simulink model "raspberrypi_sensehat_ev3robot"  (R2018b)
settings: Solver=FixedStepAuto  StartTime=0.0  StopTime=inf  RelTol=1e-3
libraries: sensehatlib x1, embdlinuxlib x1
settings Model: SimulationMode=external  Creator=The MathWorks, Inc.  LastModifiedBy=The MathWorks, Inc.
settings SolverCC: PositivePriorityOrder=on
settings OptimizationCC: MaxStackSize=64
settings DebuggingCC: ParameterTunabilityLossMsg=error
settings HardwareCC: ProdBitPerPointer=32  ProdBitPerSizeT=32  ProdBitPerPtrDiffT=32  ProdLargestAtomicInteger=Long  ProdLargestAtomicFloat=Double  ProdWordSize=32  ProdHWDeviceType=ARM Compatible->ARM Cortex  UseEmbeddedCoderFeatures=off  UseSimulinkCoderFeatures=off
settings SFSimCC: SimUseLocalCustomCode=off
settings RTWCC: SystemTargetFile=ert.tlc  HardwareBoard=Raspberry Pi  TLCOptions="-aInlineSetEventsForThisBaseRateFcn=TLC_FALSE -aSuppressMultiTaskScheduler=TLC_FALSE  -aRateBasedStepFcn=0"  TemplateMakefile=ert_default_tmf  GenerateReport=on  RTWUseLocalCustomCode=off  Toolchain=GNU GCC Raspberry Pi  LaunchReport=on
settings CodeAppCC: ForceParamTrailComments=on  OperatorAnnotations=on  StateflowObjectComments=on  MATLABSourceComments=on
settings ERTTargetCC: ERTCustomFileBanners=off  SupportContinuousTime=on  SupportNonInlinedSFcns=on  RemoveResetFunc=off  SupportVariableSizeSignals=on  ModelStepFunctionPrototypeControlCompliant=off
settings ConfigComp: CovMetricSettings=dswe

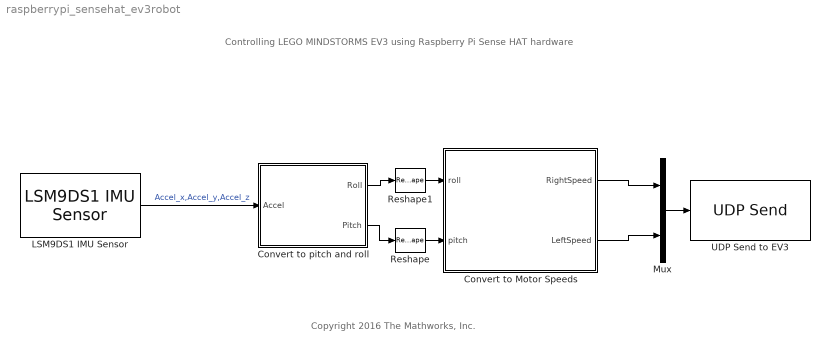
== system raspberrypi_sensehat_ev3robot ==
  note: Copyright 2016 The Mathworks, Inc.
  note: Controlling LEGO MINDSTORMS EV3
      | using
      | Raspberry Pi Sense HAT hardware
  Convert to Motor Speeds : MATLAB Function  TreatAsAtomicUnit=on
  Convert to pitch and roll : Subsystem
  LSM9DS1 IMU Sensor : sensehatlib/LSM9DS1 IMU Sensor  blockPlatform=Raspberry Pi  BoardProperty_sh=Pi 2 Model B  ActiveSensors_=Accelerometer  AccelerometerOutputDataRate=119 Hz  AccelerometerFullScaleRange=+/- 2g  AccelerometerBandwidth=50 Hz  GyroscopeOutputDataRate=119 Hz  GyroscopeFullScaleRange=245 dps  GyroscopeBandwidthMode=0  GyroscopeHighPassFilterEnabled=off  GyroscopeHighPassFilterMode=0  MagnetometerFullScaleRange=+/- 4 gauss  MagnetometerOutputDataRate=40 Hz  SampleTime=0.1
      settings: SourceProductName=Simulink Support Package for Raspberry Pi Hardware
  Mux : Mux  Inputs=2
  Reshape : Reshape  OutputDimensionality=Customize  OutputDimensions=[1]
  Reshape1 : Reshape  OutputDimensionality=Customize  OutputDimensions=[1]
  UDP Send to EV3 : embdlinuxlib/UDP Send  remoteURL='192.168.1.4'  remotePort=25000  localURL='255.255.255.255'  localPortSource=Automatically determine  localPort=-1  sampletime=-1  blockPlatform=Raspberry Pi  separateLengthPort=0
      settings: SourceProductName=Simulink Support Package for Raspberry Pi Hardware  SourceProductBaseCode=RASPPI
  wires:
  LSM9DS1 IMU Sensor/1 -> Convert to pitch and roll/1(Accel)  "Accel_x,Accel_y,Accel_z"
  Mux/1 -> UDP Send to EV3/1
  Convert to pitch and roll/1(Roll) -> Reshape1/1
  Reshape1/1 -> Convert to Motor Speeds/1(roll)
  Convert to pitch and roll/2(Pitch) -> Reshape/1
  Reshape/1 -> Convert to Motor Speeds/2(pitch)
  Convert to Motor Speeds/1(RightSpeed) -> Mux/1
  Convert to Motor Speeds/2(LeftSpeed) -> Mux/2

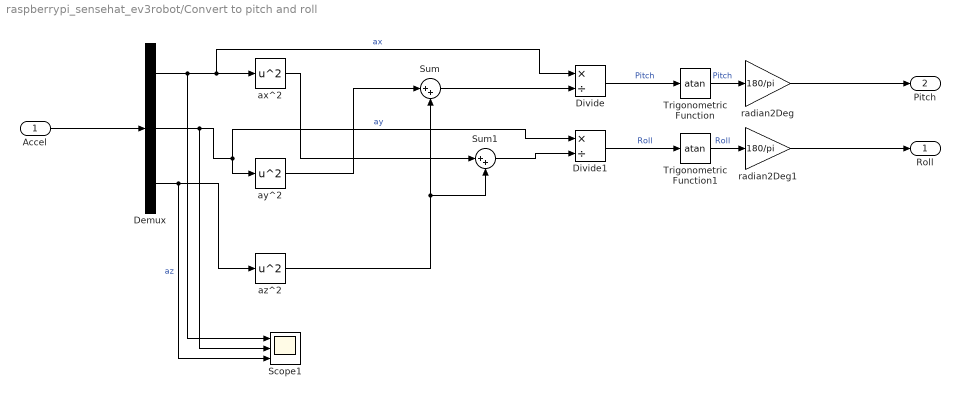
== system raspberrypi_sensehat_ev3robot/Convert to pitch and roll ==
  Accel : Inport
  Demux : Demux  Outputs=3
  Divide : Product  Inputs=*/
  Divide1 : Product  Inputs=*/
  Scope1 : Scope  NumInputPorts=3
  Sum : Sum  Inputs=|++
  Sum1 : Sum  Inputs=|++
  Trigonometric Function : Trigonometry  Operator=atan
  Trigonometric Function1 : Trigonometry  Operator=atan
  ax^2 : Math  Operator=square  SaturateOnIntegerOverflow=on
  ay^2 : Math  Operator=square  SaturateOnIntegerOverflow=on
  az^2 : Math  Operator=square  SaturateOnIntegerOverflow=on
  radian2Deg : Gain  Gain=180/pi  OutDataTypeStr=double
  radian2Deg1 : Gain  Gain=180/pi  OutDataTypeStr=double
  Roll : Outport
  Pitch : Outport  Port=2
  wires:
  Sum1/1 -> Divide1/2
  Sum/1 -> Divide/2
  ax^2/1 -> Sum1/1
  Demux/1 -> Scope1/1, Divide/1, ax^2/1  "ax"
  Demux/3 -> Scope1/3, az^2/1  "az"
  Divide/1 -> Trigonometric Function/1  "Pitch"
  az^2/1 -> Sum1/2, Sum/2
  ay^2/1 -> Sum/1
  Trigonometric Function1/1 -> radian2Deg1/1  "Roll"
  Trigonometric Function/1 -> radian2Deg/1  "Pitch"
  Divide1/1 -> Trigonometric Function1/1  "Roll"
  Accel/1 -> Demux/1
  Demux/2 -> Scope1/2, Divide1/1, ay^2/1  "ay"
  radian2Deg/1 -> Pitch/1
  radian2Deg1/1 -> Roll/1

== matlab function raspberrypi_sensehat_ev3robot/Convert to Motor Speeds ==
  data: RightSpeed output; LeftSpeed output; roll input; pitch input
function [RightSpeed,LeftSpeed]= roll_pitch_to_speed(roll,pitch)

% The input is the Sense Hat Roll and Pitch angles.
% Output is the Left wheel velocity (Vl) and Right wheel Velocity (Vr).
% The output to the wheel varies from -100 for Full power reverse to 100
% for Full power forward

%% Robot Parameters
len = 15;
% Distance between the two wheels of Lego EV3 robot in centimeters

v_max = 100;
% The maximum possible linear speed of the Robot, equal to
% (Vl_max + Vr_max)/2 = (100 + 100)/2 = 100;

w_max = 200/len;
% The maximum possible angular speed of the Robot, equal to
% (Vl_max - Vl_min)/len = (100 - (-100))/len = 200/len

% Initialize variables
v = 0;
omega = 0;
% The robot should not move in its default state


%% Calculate the Angular Velocity of the Robot
if (abs(pitch) <= 2)
    omega = 0;
    % For very small input, do not rotate the robot
end


if (pitch >2 && pitch <= 40)
    omega = w_max*(0.2*(pitch - 2)/38);
    % at 2 --> omega = 0, at 40 --> omega = 0.2*w_max
end

if (pitch <-2 && pitch >= -40)
    omega = w_max*(0.2*(pitch + 2)/38);
    % at -2 --> omega = 0, at -40 --> omega = -0.2*w_max
end


if (pitch >40 && pitch <= 70)
    omega = w_max*(0.01*pitch - 0.2);
    % at 40 --> omega = 0.2*w_max, at 70 --> omega = 0.5*w_max
end

if (pitch <- 40 && pitch >= -70)
    omega = w_max*(0.01*pitch + 0.2);
    % at -40 --> omega = -0.2*w_max, at -70 --> omega = -0.5*w_max
end


if (pitch> 70)
    omega = w_max*0.5;
    % Saturate omega to 0.5*w_max, since it is very difficult to control
    % the EV3 rotating faster than 0.5*w_max
end

if (pitch < -70)
    omega = -w_max*0.5;
    % Saturate |omega| to 0.5*w_max
end

if (abs(roll) <= 5)
    v = 0;
    % For very small input, do not move the robot
end

% The angular veloctiy (omega) is saturated to 0.5 times the maximum
% angular velocity (w_max), since it is very difficult to control the robot
% rotating faster than 0.5*w_max

%% Calculate the Linear Velocity of the Robot
if (roll > 5 && roll <= 60)
    v = v_max*(0.9*(roll - 5)/55);
    % at 5 --> v = 0, at 60 --> v = 0.9*v_max
end

if (roll < -5 && roll >= -60)
    v = v_max*(0.9*(roll + 5)/55);
    % at -5 --> v = 0, at -60 --> v = -0.9*v_max
end

if (roll > 60)
    v = v_max*0.9;
    % Saturate v to 0.9*v_max
end

if (roll < -60)
    v = -v_max*0.9;
    % Saturate |v| to 0.9*v_max
end

% The velocity (v) is saturated to 0.9 times the maximum linear velocity
% for the robot (v_max), to give room for the robot to turn as it is moving
% forward. If the maximum velocity is set to v_max, the output for both the
% wheels is saturated to 100, and the robot cannot turn.

%% Differential Drive Robot equations
% When the robot is moving forwards
if (v >= 0)
    Vr = v + omega*len/2;
    Vl = v - omega*len/2;
else % robot is moving in reverse
    Vr = v - omega*len/2;
    Vl = v + omega*len/2;
end
% V is the linear velocity of the robot, omega is the angular velocity of
% the robot, and len is the distance between the two wheels of the robot

%% Sautrate the |output| to 100, the limit of the LEGO EV3 motor block
if (Vl > 100)
    Vl = 100;
end

if (Vl < -100)
    Vl = -100;
end

if (Vr > 100)
    Vr = 100;
end

if (Vr < -100)
    Vr = -100;
end

%% Convert to int8 since the Lego EV3 block accepts integers
LeftSpeed = int8(Vl);
RightSpeed = int8(Vr);

end
